simulink model "Juneanalysis"  (R2025a)
settings: Solver=VariableStepAuto  StartTime=0.0  StopTime=130  RelTol=1e-3
libraries: spsSeriesRLCBranchLib x4, spsDiodeLib x1, spsIGBTDiodeLib x1, spsMosfetLib x1, spsPVArrayLib x1, spsPWMGeneratorDCDCLib x1, sps_lib x1
settings Model: Creator=Jawwad  LastModifiedBy=Jawwad

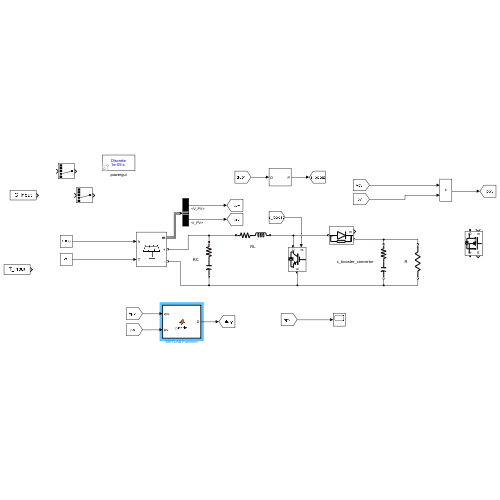
[thumbnail: Simulink's stored preview of the top-level diagram]
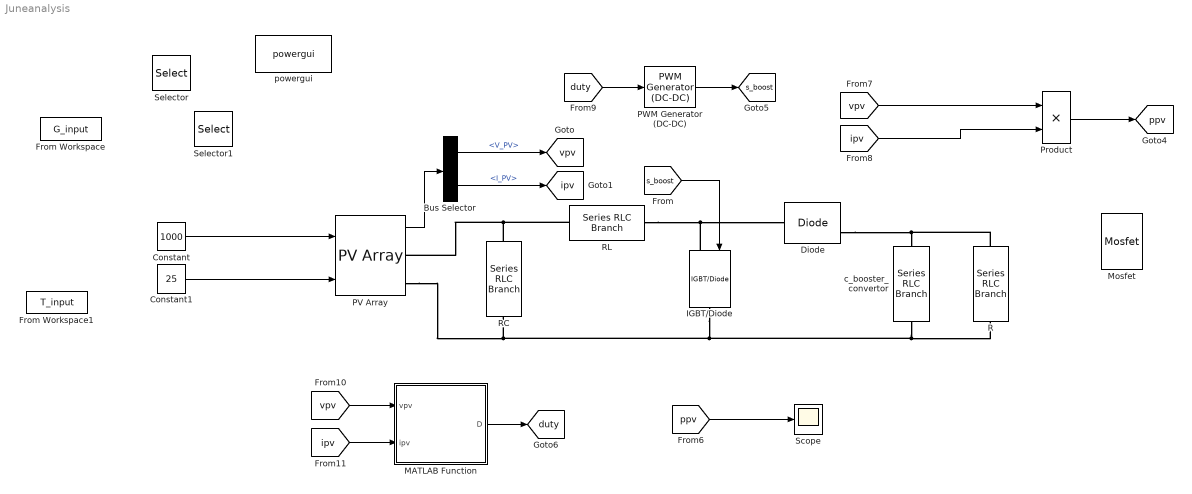
== system Juneanalysis ==
  Bus Selector : BusSelector  OutputSignals=V_PV,I_PV
  Constant : Constant  Value=1000
  Constant1 : Constant  Value=25
  Diode : spsDiodeLib/Diode  Ron=0.001  Lon=0  Vf=0.8  IC=0  UseSnubber=0  Rs=500  Cs=250e-9  Measurements=on
  From Workspace : FromWorkspace  VariableName=G_input
  From Workspace1 : FromWorkspace  VariableName=T_input
  IGBT/Diode : spsIGBTDiodeLib/IGBT//Diode  Ron=1e-3  Rs=1e5  Cs=inf  Measurements=off
  MATLAB Function : MATLAB Function  TreatAsAtomicUnit=on
  Mosfet : spsMosfetLib/Mosfet  Ron=0.1  Lon=0  Rd=0.01  Vfd=0  IC=0  Rs=1e5  Cs=inf  Measurements=on
  PV Array : spsPVArrayLib/PV Array  Npar=1  Nser=1  PlotType=array @ 1000 W/m2 & specified temperatures  S_vec="[ 1000  500  100 ]"  Temp_C_vec="[ 45 25  ]"  ModuleName=User-defined  PlotWhenSelected=off  Pm=213.15  Ncell=60  Voc=36.3  Isc=7.84  Vm=29  Im=7.35  beta_Voc_pc=-0.36099  alpha_Isc_pc=0.102  beta_Voc=-0.13104  alpha_Isc=0.0079968  IL=7.8654  I0=2.9273e-10  nI=0.98119  Rsh=313.0553  Rs=0.39381  RobustModel=off  RobustCellTemperature=313.3991  BAL=on  Tc=1e-6  Tfilter=5e-5
  PWM Generator (DC-DC) : spsPWMGeneratorDCDCLib/PWM Generator (DC-DC)  Fsw=5000  Ts=10e-6
  Product : Product
  R : spsSeriesRLCBranchLib/Series RLC Branch  LConnTagsString=__new0  RConnTagsString=__new0  BranchType=R  Resistance=10  Inductance=1e-3  SetiL0=off  InitialCurrent=0  Capacitance=100e-6  Setx0=off  InitialVoltage=0  Measurements=None
  RC : spsSeriesRLCBranchLib/Series RLC Branch  LConnTagsString=__new0  RConnTagsString=__new0  BranchType=RC  Resistance=1e-4  Inductance=1e-3  SetiL0=off  InitialCurrent=0  Capacitance=100e-6  Setx0=off  InitialVoltage=0  Measurements=None
  RL : spsSeriesRLCBranchLib/Series RLC Branch  LConnTagsString=__new0  RConnTagsString=__new0  BranchType=RL  Resistance=0.1  Inductance=5e-3  SetiL0=off  InitialCurrent=0  Capacitance=1e-6  Setx0=off  InitialVoltage=0  Measurements=None
  Scope : Scope
      settings: ActiveDisplayYMinimum=-141.38577509649576  ActiveDisplayYMaximum=261.05219795390678
  Selector : Selector  InputPortWidth=5  IndexOptions=Index vector (dialog)  Indices=[4]  OutputSizes=1
  Selector1 : Selector  InputPortWidth=5  IndexOptions=Index vector (dialog)  Indices=[4]  OutputSizes=1
  c_booster_convertor : spsSeriesRLCBranchLib/Series RLC Branch  LConnTagsString=__new0  RConnTagsString=__new0  BranchType=RC  Resistance=1e-4  Inductance=1e-3  SetiL0=off  InitialCurrent=0  Capacitance=100e-6  Setx0=off  InitialVoltage=0  Measurements=None
  powergui : sps_lib/powergui  Priority=1  SimulationMode=Discrete  SampleTime=1e-5  frequency=60  Iterations=50  frequencyindice=0  Pbase=100e6  ErrMax=1e-4  UnitsV=kV  UnitsW=MW  buscounter=0  FunctionMessages=off  echomessages=off  EnableUseOfTLC=off  CurrentSourceSwitches=off  DisableSnubberDevices=off  DisableRonSwitches=off  DisableVfSwitches=off  DisplayEquations=off  AutomaticDiscreteSolvers=off  SolverType=Tustin/Backward Euler (TBE)  Interpol=off  ExternalGateDelay=off  methode=off  Ts=100  x0status=blocks  SPID=on  SwTol=0  HookPort=off  NonlinearTolerance=1e-4  nMaxIteration=100  ContinueOnMaxIteration=off  RestoreLinks=warning  ResistiveCurrentMeasurement=off  Frange=[0:2:500]  Ylog=off  Xlog=on  ShowGrid=off  save=off  variable=ZData  structure=0  ZoomFFT=off  StartTime=0.0  cycles=1  DisplayStyle=1  fundamental=60  FreqAxis=off  MaxFrequency=1000  frequencyindicesteady=1  RmsSteady=1  display=off
  tag scope: duty=global, ipv=global, ppv=global, s_boost=global, vpv=global
  wires:
  Bus Selector/2 -> [ipv]  "<I_PV>"
  [vpv] -> Product/1
  MATLAB Function/1(D) -> [duty]
  Product/1 -> [ppv]
  [vpv] -> MATLAB Function/1(vpv)
  Bus Selector/1 -> [vpv]  "<V_PV>"
  [ipv] -> Product/2
  PV Array/1 -> Bus Selector/1
  PWM Generator (DC-DC)/1 -> [s_boost]
  [ppv] -> Scope/1
  [duty] -> PWM Generator (DC-DC)/1
  [ipv] -> MATLAB Function/2(ipv)
  [s_boost] -> IGBT/Diode/1
  Constant/1 -> PV Array/1
  Constant1/1 -> PV Array/2
  connections:
  RL/RConn1 -- Diode/LConn1 -- IGBT/Diode/LConn1
  c_booster_convertor/LConn1 -- Diode/RConn1 -- R/LConn1
  c_booster_convertor/RConn1 -- IGBT/Diode/RConn1 -- PV Array/RConn2 -- RC/RConn1 -- R/RConn1
  PV Array/RConn1 -- RC/LConn1 -- RL/LConn1

== matlab function Juneanalysis/MATLAB Function ==
  data: vpv input; D output; ipv input
function D = pando(vpv, ipv)
    % PERSISTENT variables to store history between simulation steps
    persistent Dprev Vprev Pprev
    
    % Initialize if it's the first run
    if isempty(Dprev)
        Dprev = 0.7;
        Vprev = 190;   % Start from 0 to allow initial ramp-up
        Pprev = 2000;
    end
    
    % Step size (Adjust based on your converter's sensitivity)
    deltaD = 125e-6; % 125e-6 is very small; might take long to reach MPP
    
    % Calculate current power
    ppv = vpv * ipv;
    
    % P&O Logic
    deltaP = ppv - Pprev;
    deltaV = vpv - Vprev;
    
    if deltaP ~= 0
        if deltaP > 0
            if deltaV > 0
                % Power increasing and Voltage increasing: Move left (decrease D)
                D = Dprev - deltaD;
            else
                % Power increasing and Voltage decreasing: Move right (increase D)
                D = Dprev + deltaD;
            end
        else
            if deltaV > 0
                % Power decreasing and Voltage increasing: Move right (increase D)
                D = Dprev + deltaD;
            else
                % Power decreasing and Voltage decreasing: Move left (decrease D)
                D = Dprev - deltaD;
            end
        end
    else
        D = Dprev;
    end
    
    % --- CRITICAL FIX: Limit Duty Cycle (0 to 1) ---
    if D > 0.9
        D = 0.9;
    elseif D < 0.1
        D = 0.1;
    end
    
    % --- CRITICAL FIX: Update state for the next step ---
    Dprev = D;
    Vprev = vpv;
    Pprev = ppv;
end
